simulink model "poleplace_luenburg_foo"  (Simulink 7.5)
settings: Solver=ode4  StartTime=0.0  StopTime=13.5  FixedStep=0.001  RelTol=1e-3
PreLoadFcn:
  | poleplace_luenburg_foo_param
values from neighbouring files (symbols this model uses):
  A = [0  -20.6; 1 0],    [poleplace_luenburg_foo_param.m]    (also in poleplace_luenburg_roo_param.m = [0  1  0; 0  0  1; 0  0  0],; poleplace_sfb_luenburg_foo_param.m = [0  1; 0  -5],; poleplace_sfb_luenburg_roo_param.m = [0  1  0; 0  0  1; -6  -11  -6],)
  B = [0; 1],    [poleplace_luenburg_foo_param.m]    (also in poleplace_luenburg_roo_param.m = [0; 0; 1],; poleplace_sfb_luenburg_foo_param.m = [0; 100],; poleplace_sfb_luenburg_roo_param.m = [0; 0; 1],)
  C = [0 1],    [poleplace_luenburg_foo_param.m]    (also in poleplace_luenburg_roo_param.m = [1 0 0],; poleplace_sfb_luenburg_foo_param.m = [1 0],; poleplace_sfb_luenburg_roo_param.m = [1 0 0],)
  G = phi_A*inv(N)*[0; 1]    [poleplace_luenburg_foo_param.m]    (also in poleplace_luenburg_roo_param.m = acker(A11', A21',  pole_esti_desired )',; poleplace_sfb_luenburg_foo_param.m = acker(A', C', p)'; poleplace_sfb_luenburg_roo_param.m = acker(Abb', Aab',  pole_esti_desired )',)
libraries: simulink x2
settings Model: Creator=Huiliang  LastModifiedBy=Dell
settings OptimizationCC: InitFltsAndDblsToZero=on
settings DebuggingCC: SaveWithParameterizedLinksMsg=none  StrictBusMsg=Warning
settings GRTTargetCC: TargetFcnLib=ansi_tfl_tmw.mat

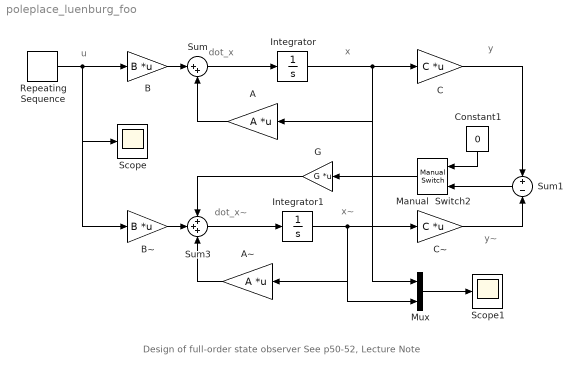
== system poleplace_luenburg_foo ==
  note: x
  note: dot_x
  note: y
  note: u
  note: x~
  note: dot_x~
  note: y~
  note: Design of full-order state observer
      | See p50-52, Lecture Note
  A : Gain  Gain=A  Multiplication=Matrix(K*u)  ParameterDataType=sfix(16)  ParameterScaling=2^0  OutDataType=sfix(16)  OutScaling=2^0
  A~ : Gain  Gain=A  Multiplication=Matrix(K*u)  ParameterDataType=sfix(16)  ParameterScaling=2^0  OutDataType=sfix(16)  OutScaling=2^0
  B : Gain  Gain=B  Multiplication=Matrix(K*u)  ParameterDataType=sfix(16)  ParameterScaling=2^0  OutDataType=sfix(16)  OutScaling=2^0
  B~ : Gain  Gain=B  Multiplication=Matrix(K*u)  ParameterDataType=sfix(16)  ParameterScaling=2^0  OutDataType=sfix(16)  OutScaling=2^0
  C : Gain  Gain=C  Multiplication=Matrix(K*u)  ParameterDataType=sfix(16)  ParameterScaling=2^0  OutDataType=sfix(16)  OutScaling=2^0
  Constant1 : Constant  Value=0  OutDataType=fixdt(1, 16)  OutScaling=2^0
  C~ : Gain  Gain=C  Multiplication=Matrix(K*u)  ParameterDataType=sfix(16)  ParameterScaling=2^0  OutDataType=sfix(16)  OutScaling=2^0
  G : Gain  Gain=G  Multiplication=Matrix(K*u)  ParameterDataType=sfix(16)  ParameterScaling=2^0  OutDataType=sfix(16)  OutScaling=2^0
  Integrator : Integrator  InitialCondition="[0.2;  -0.2]"
  Integrator1 : Integrator  InitialCondition="[0;    0]"
  Manual  Switch2 : simulink/Signal Routing/Manual Switch  SystemSampleTime=-1  sw=0  action=0  varsize=off
  Mux : Mux  Inputs=2
  Repeating Sequence : simulink/Sources/Repeating Sequence  SystemSampleTime=-1  rep_seq_t="[0  3  3  3.5]"  rep_seq_y="[0  0  1  1]"
  Scope : Scope
      settings: TimeRange=14  YMin=-0.5  YMax=1.5  MaxDataPoints=50000
  Scope1 : Scope
      settings: TimeRange=14  YMin=-2  YMax=2  MaxDataPoints=500000
  Sum : Sum  Inputs=|++  OutDataType=sfix(16)  OutScaling=2^0
  Sum1 : Sum  Inputs=+|-  OutDataType=sfix(16)  OutScaling=2^0
  Sum3 : Sum  Inputs=+++  OutDataType=sfix(16)  OutScaling=2^0
  wires:
  Integrator/1 -> A/1, C/1, Mux/1
  C/1 -> Sum1/1
  Sum/1 -> Integrator/1
  A/1 -> Sum/2
  B/1 -> Sum/1
  Integrator1/1 -> C~/1, A~/1, Mux/2
  Sum3/1 -> Integrator1/1
  Repeating Sequence/1 -> B/1, B~/1, Scope/1
  B~/1 -> Sum3/2
  G/1 -> Sum3/1
  C~/1 -> Sum1/2
  A~/1 -> Sum3/3
  Mux/1 -> Scope1/1
  Manual  Switch2/1 -> G/1
  Sum1/1 -> Manual  Switch2/2
  Constant1/1 -> Manual  Switch2/1
